simulink model "timeSharedS"  (R2023a)
settings: Solver=VariableStepAuto  StartTime=0.0  StopTime=10.0  RelTol=1e-3
libraries: NSA_DEVS_SINKS_ATOMIC x6, NSA_DEVS_LOGISTICS_ATOMIC x3, TimeSharedLib x2, NSA_DEVS_ROUTING_ATOMIC x2, NSA_DEVS_SOURCES_ATOMIC x1, NSA_DEVS_MATH_OPERATIONS_ATOMIC x1
settings Model: Creator=peter  LastModifiedBy=peter

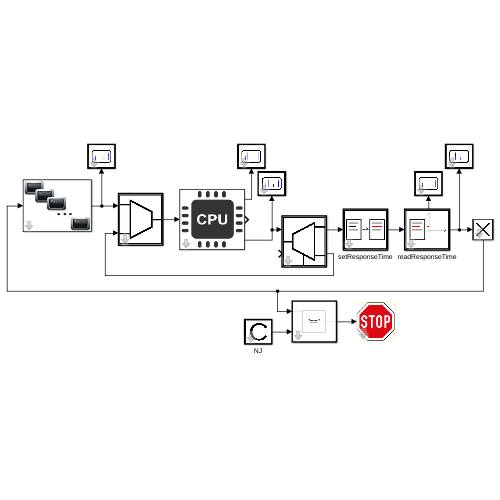
[thumbnail: Simulink's stored preview of the top-level diagram]
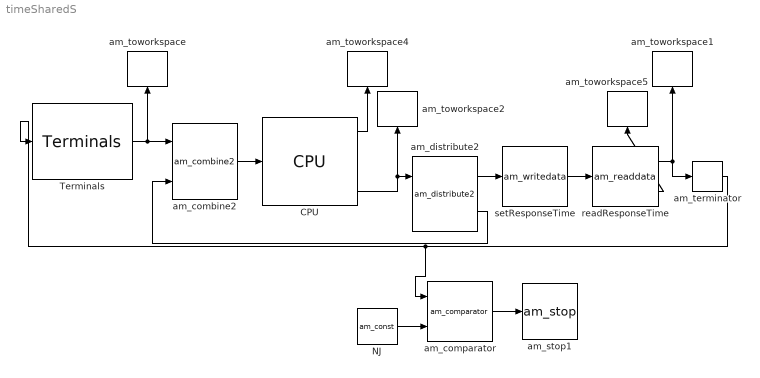
== system timeSharedS ==
  CPU : TimeSharedLib/CPU  q=1  tSwap=0.1
  NJ : NSA_DEVS_SOURCES_ATOMIC/am_const  value=10  sendTime=[0,1]  tau=[0,1]  debug=0
      settings: SourceProductName=NSA_DEVS
  Terminals : TimeSharedLib/Terminals  N=3  tW=7  tS=5
  am_combine2 : NSA_DEVS_ROUTING_ATOMIC/am_combine2  tD=[0,2]  tau=[0,1]  debug=0
      settings: SourceProductName=NSA_DEVS
  am_comparator : NSA_DEVS_MATH_OPERATIONS_ATOMIC/am_comparator  compop="\"==\""  tau=[0,1]  debug=0
      settings: SourceProductName=NSA_DEVS
  am_distribute2 : NSA_DEVS_ROUTING_ATOMIC/am_distribute2  port0=1  field="\"outPort\""  tau=[0,1]  debug=0
      settings: SourceProductName=NSA_DEVS
  am_stop1 : NSA_DEVS_SINKS_ATOMIC/am_stop  tau=[0,1]  debug=0
      settings: SourceProductName=NSA_DEVS
  am_terminator : NSA_DEVS_LOGISTICS_ATOMIC/am_terminator  tau=[0,1]  debug=0
      settings: SourceProductName=NSA_DEVS
  am_toworkspace : NSA_DEVS_SINKS_ATOMIC/am_toworkspace  varname="\"termOut\""  t0=0  format="\"vector\""  tau=[0,1]  debug=0
      settings: SourceProductName=NSA_DEVS
  am_toworkspace1 : NSA_DEVS_SINKS_ATOMIC/am_toworkspace  varname="\"jobsOut\""  t0=0  format="\"vector\""  tau=[0,1]  debug=0
      settings: SourceProductName=NSA_DEVS
  am_toworkspace2 : NSA_DEVS_SINKS_ATOMIC/am_toworkspace  varname="\"cpuOut\""  t0=0  format="\"vector\""  tau=[0,1]  debug=0
      settings: SourceProductName=NSA_DEVS
  am_toworkspace4 : NSA_DEVS_SINKS_ATOMIC/am_toworkspace  varname="\"nQ\""  t0=0  format="\"vector\""  tau=[0,5]  debug=0
      settings: SourceProductName=NSA_DEVS
  am_toworkspace5 : NSA_DEVS_SINKS_ATOMIC/am_toworkspace  varname="\"timeOut\""  t0=0  format="\"vector\""  tau=[0,1]  debug=0
      settings: SourceProductName=NSA_DEVS
  readResponseTime : NSA_DEVS_LOGISTICS_ATOMIC/am_readdata  field="\"startTime\""  tau=[0,1]  debug=0
      settings: SourceProductName=NSA_DEVS
  setResponseTime : NSA_DEVS_LOGISTICS_ATOMIC/am_writedata  inFields="\"startTime\""  outField="\"startTime\""  changeFunc="\"out = get_time() - in(1);\""  tau=[0,1]  debug=0
      settings: SourceProductName=NSA_DEVS
  wires:
  Terminals/1 -> am_combine2/1, am_toworkspace/1
  am_combine2/1 -> CPU/1
  CPU/3 -> am_distribute2/1, am_toworkspace2/1
  am_distribute2/1 -> setResponseTime/1
  am_terminator/1 -> am_comparator/1, Terminals/1
  CPU/1 -> am_toworkspace4/1
  am_comparator/1 -> am_stop1/1
  NJ/1 -> am_comparator/2
  readResponseTime/1 -> am_terminator/1, am_toworkspace1/1
  readResponseTime/2 -> am_toworkspace5/1
  setResponseTime/1 -> readResponseTime/1
  am_distribute2/2 -> am_combine2/2
